simulink model "env_mdl_aero_blockset"  (R2020b)
settings: Solver=VariableStepAuto  StartTime=0.0  StopTime=10.0  RelTol=1e-3
undefined symbols (not defined in the file): decyear, now, WMM2020
libraries: aerolibconvert2 x2, aerolibgravity2 x2, aerolibatmos2 x1
settings Model: Creator=brian  LastModifiedBy=brian

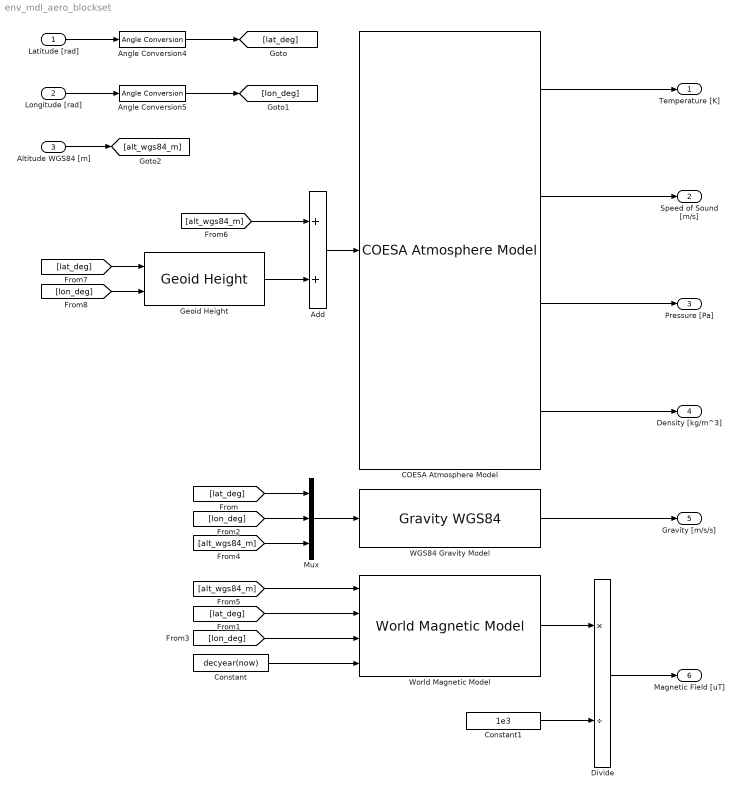
== system env_mdl_aero_blockset ==
  Latitude [rad] : Inport
  Longitude [rad] : Inport  Port=2
  Altitude WGS84 [m] : Inport  Port=3
  Add : Sum
  Angle Conversion4 : aerolibconvert2/Angle Conversion  IU=rad  OU=deg
  Angle Conversion5 : aerolibconvert2/Angle Conversion  IU=rad  OU=deg
  COESA Atmosphere Model : aerolibatmos2/COESA Atmosphere Model  units=Metric (MKS)  spec=1976 COESA-extended U.S. Standard Atmosphere  model=Profile  profile_var=High temperature  profile_percent=1%  profile_alt=5 km (16404 ft)  envelope_var=High temperature  envelope_percent=1%  action=Warning
  Constant : Constant  Value=decyear(now)
  Constant1 : Constant  Value=1e3
  Divide : Product  Inputs=*/
  Geoid Height : aerolibgravity2/Geoid Height  units=Metric (MKS)  gtype=EGM2008  datafile='geoidegm96grid'  dtype=double  action=Warning
      settings: SourceProductBaseCode=AE
  Mux : Mux  Inputs=3
  "WGS84 Gravity Model  " : GravityWGS84
  World Magnetic Model : aerolibgravity2/World Magnetic Model  model=WMM2020 (2020-2025)  customFile='WMM2020.COF'  units=Metric (MKS)  time_in=on  month=January  day=1  year=2020  action=Error  h_out=off  dec_out=off  inc_out=off  ti_out=off
      settings: SourceProductBaseCode=AE
  Temperature [K] : Outport
  Speed of Sound [m/s] : Outport  Port=2
  Pressure [Pa] : Outport  Port=3
  Density [kg/m^3] : Outport  Port=4
  Gravity [m/s/s] : Outport  Port=5
  Magnetic Field [uT] : Outport  Port=6
  wires:
  [lon_deg] -> Mux/2
  Mux/1 -> "WGS84 Gravity Model  "/1
  [lon_deg] -> World Magnetic Model/3
  Constant/1 -> World Magnetic Model/4
  [lat_deg] -> Mux/1
  [lat_deg] -> World Magnetic Model/2
  Altitude WGS84 [m]/1 -> [alt_wgs84_m]
  [alt_wgs84_m] -> Mux/3
  [alt_wgs84_m] -> World Magnetic Model/1
  Angle Conversion4/1 -> [lat_deg]
  Latitude [rad]/1 -> Angle Conversion4/1
  Angle Conversion5/1 -> [lon_deg]
  Longitude [rad]/1 -> Angle Conversion5/1
  Add/1 -> COESA Atmosphere Model/1
  Geoid Height/1 -> Add/2
  [alt_wgs84_m] -> Add/1
  [lat_deg] -> Geoid Height/1
  [lon_deg] -> Geoid Height/2
  Divide/1 -> Magnetic Field [uT]/1
  World Magnetic Model/1 -> Divide/1
  "WGS84 Gravity Model  "/1 -> Gravity [m/s/s]/1
  COESA Atmosphere Model/4 -> Density [kg/m^3]/1
  COESA Atmosphere Model/3 -> Pressure [Pa]/1
  COESA Atmosphere Model/2 -> Speed of Sound [m/s]/1
  COESA Atmosphere Model/1 -> Temperature [K]/1
  Constant1/1 -> Divide/2
